simulink model "Simulink_serial_example"  (Simulink 8.8)
settings: Solver=FixedStepDiscrete  StartTime=0.0  StopTime=50  RelTol=1e-3  EnableMultiTasking=on
undefined symbols (not defined in the file or in its folder): fdesignblkfcn, gcbh, serial
libraries: instrumentlib x2
settings Model: Creator=skolak  LastModifiedBy=qhsam
settings OptimizationCC: InitFltsAndDblsToZero=on
settings DebuggingCC: SaveWithParameterizedLinksMsg=none  SignalResolutionControl=TryResolveAllWithWarning  SolverPrmCheckMsg=warning  MultiTaskDSMMsg=warning  MultiTaskCondExecSysMsg=none  StateNameClashWarn=none
settings GRTTargetCC: TargetFcnLib=ansi_tfl_tmw.mat  GeneratePreprocessorConditionals=Use local settings

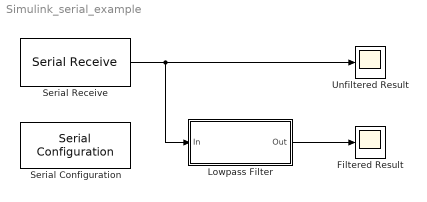
== system Simulink_serial_example ==
  Filtered Result : Scope
  Lowpass Filter : Subsystem  DialogController=fdesignblkfcn  DialogControllerArgs=DataTag1  InitFcn=fdesignblkfcn(gcbh, {'InitFcn'});  mask(Lowpass Filter){}
      mask help: Design a lowpass filter
      settings: CopyFcn=fdesignblkfcn(gcbh, {'CopyFcn'});
      mask Help: helpview(mapfilelocation('dspblks'), 'dsplowpassfilter')
      mask Display: disp('Lowpass')
  Serial Configuration : instrumentlib/Serial Configuration  Priority=-200000  ComPortMenu=COM5  ComPort=COM5  ObjConstructor=serial('COM5');  BaudRate=9600  DataBits=8  Parity=none  StopBits=1  FlowControl=none  Timeout=10  ByteOrder=LittleEndian
  Serial Receive : instrumentlib/Serial Receive  ComPortMenu=COM5  ComPort=COM5  ObjConstructor=serial('COM5');  Terminator=<none>  DataSize=[1 1]  DataType=uint8  EnableBlockingMode=on  ActionDataUnavailable=Output last received value  CustomValue=0  SampleTime=0.01
  Unfiltered Result : Scope
  wires:
  Lowpass Filter/1(Out) -> Filtered Result/1
  Serial Receive/1 -> Lowpass Filter/1(In), Unfiltered Result/1

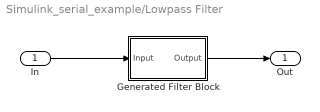
== system Simulink_serial_example/Lowpass Filter ==
  In : Inport
  Generated Filter Block : Subsystem  Tag=FilterWizardSubSystem
      settings: ErrorFcn=dspFilterRealizedInBasicElemsAlgLoopErrFcnCallback
  Out : Outport
  wires:
  In/1 -> Generated Filter Block/1(Input)
  Generated Filter Block/1(Output) -> Out/1

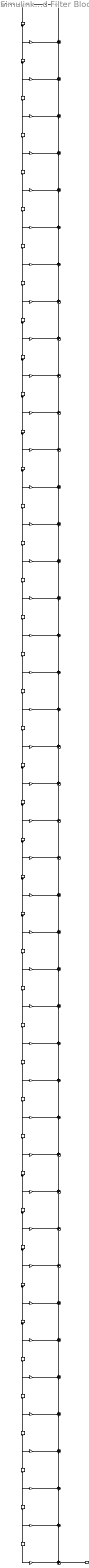
== system Simulink_serial_example/Lowpass Filter/Generated Filter Block ==
  Input : Inport
  BodyDelay{2..43} (42 alike) : Delay  DelayLength=1  InitialCondition=0  InputProcessing=Inherited
  BodyLSum{2..43} (42 alike) : Sum  Inputs=++|  RndMeth=Nearest  SaturateOnIntegerOverflow=on  OutDataTypeStr=Inherit: Same as first input
  b(1) : Gain  Gain=-0.002422873852326935  ParamDataTypeStr=double  RndMeth=Nearest  SaturateOnIntegerOverflow=on  OutDataTypeStr=Inherit: Same as input
  b(10) : Gain  Gain=-0.010121234703278952  ParamDataTypeStr=double  RndMeth=Nearest  SaturateOnIntegerOverflow=on  OutDataTypeStr=Inherit: Same as input
  b(11) : Gain  Gain=-0.018273518733782461  ParamDataTypeStr=double  RndMeth=Nearest  SaturateOnIntegerOverflow=on  OutDataTypeStr=Inherit: Same as input
  b(12) : Gain  Gain=0.011431962071777995  ParamDataTypeStr=double  RndMeth=Nearest  SaturateOnIntegerOverflow=on  OutDataTypeStr=Inherit: Same as input
  b(13) : Gain  Gain=0.026175888580407654  ParamDataTypeStr=double  RndMeth=Nearest  SaturateOnIntegerOverflow=on  OutDataTypeStr=Inherit: Same as input
  b(14) : Gain  Gain=-0.012489027835322949  ParamDataTypeStr=double  RndMeth=Nearest  SaturateOnIntegerOverflow=on  OutDataTypeStr=Inherit: Same as input
  b(15) : Gain  Gain=-0.037996623145463641  ParamDataTypeStr=double  RndMeth=Nearest  SaturateOnIntegerOverflow=on  OutDataTypeStr=Inherit: Same as input
  b(16) : Gain  Gain=0.013388945199366911  ParamDataTypeStr=double  RndMeth=Nearest  SaturateOnIntegerOverflow=on  OutDataTypeStr=Inherit: Same as input
  b(17) : Gain  Gain=0.05815546581472987  ParamDataTypeStr=double  RndMeth=Nearest  SaturateOnIntegerOverflow=on  OutDataTypeStr=Inherit: Same as input
  b(18) : Gain  Gain=-0.014048043515808944  ParamDataTypeStr=double  RndMeth=Nearest  SaturateOnIntegerOverflow=on  OutDataTypeStr=Inherit: Same as input
  b(19) : Gain  Gain=-0.10272466857882172  ParamDataTypeStr=double  RndMeth=Nearest  SaturateOnIntegerOverflow=on  OutDataTypeStr=Inherit: Same as input
  b(2) : Gain  Gain=-0.0020832449820792948  ParamDataTypeStr=double  RndMeth=Nearest  SaturateOnIntegerOverflow=on  OutDataTypeStr=Inherit: Same as input
  b(20) : Gain  Gain=0.014462275771238391  ParamDataTypeStr=double  RndMeth=Nearest  SaturateOnIntegerOverflow=on  OutDataTypeStr=Inherit: Same as input
  b(21) : Gain  Gain=0.31716649721769491  ParamDataTypeStr=double  RndMeth=Nearest  SaturateOnIntegerOverflow=on  OutDataTypeStr=Inherit: Same as input
  b(22) : Gain  Gain=0.48538764678732516  ParamDataTypeStr=double  RndMeth=Nearest  SaturateOnIntegerOverflow=on  OutDataTypeStr=Inherit: Same as input
  b(23) : Gain  Gain=0.31716649721769491  ParamDataTypeStr=double  RndMeth=Nearest  SaturateOnIntegerOverflow=on  OutDataTypeStr=Inherit: Same as input
  b(24) : Gain  Gain=0.014462275771238391  ParamDataTypeStr=double  RndMeth=Nearest  SaturateOnIntegerOverflow=on  OutDataTypeStr=Inherit: Same as input
  b(25) : Gain  Gain=-0.10272466857882172  ParamDataTypeStr=double  RndMeth=Nearest  SaturateOnIntegerOverflow=on  OutDataTypeStr=Inherit: Same as input
  b(26) : Gain  Gain=-0.014048043515808944  ParamDataTypeStr=double  RndMeth=Nearest  SaturateOnIntegerOverflow=on  OutDataTypeStr=Inherit: Same as input
  b(27) : Gain  Gain=0.05815546581472987  ParamDataTypeStr=double  RndMeth=Nearest  SaturateOnIntegerOverflow=on  OutDataTypeStr=Inherit: Same as input
  b(28) : Gain  Gain=0.013388945199366911  ParamDataTypeStr=double  RndMeth=Nearest  SaturateOnIntegerOverflow=on  OutDataTypeStr=Inherit: Same as input
  b(29) : Gain  Gain=-0.037996623145463641  ParamDataTypeStr=double  RndMeth=Nearest  SaturateOnIntegerOverflow=on  OutDataTypeStr=Inherit: Same as input
  b(3) : Gain  Gain=0.0067703446401186605  ParamDataTypeStr=double  RndMeth=Nearest  SaturateOnIntegerOverflow=on  OutDataTypeStr=Inherit: Same as input
  b(30) : Gain  Gain=-0.012489027835322949  ParamDataTypeStr=double  RndMeth=Nearest  SaturateOnIntegerOverflow=on  OutDataTypeStr=Inherit: Same as input
  b(31) : Gain  Gain=0.026175888580407654  ParamDataTypeStr=double  RndMeth=Nearest  SaturateOnIntegerOverflow=on  OutDataTypeStr=Inherit: Same as input
  b(32) : Gain  Gain=0.011431962071777995  ParamDataTypeStr=double  RndMeth=Nearest  SaturateOnIntegerOverflow=on  OutDataTypeStr=Inherit: Same as input
  b(33) : Gain  Gain=-0.018273518733782461  ParamDataTypeStr=double  RndMeth=Nearest  SaturateOnIntegerOverflow=on  OutDataTypeStr=Inherit: Same as input
  b(34) : Gain  Gain=-0.010121234703278952  ParamDataTypeStr=double  RndMeth=Nearest  SaturateOnIntegerOverflow=on  OutDataTypeStr=Inherit: Same as input
  b(35) : Gain  Gain=0.012982883808855773  ParamDataTypeStr=double  RndMeth=Nearest  SaturateOnIntegerOverflow=on  OutDataTypeStr=Inherit: Same as input
  b(36) : Gain  Gain=0.0092567976151380332  ParamDataTypeStr=double  RndMeth=Nearest  SaturateOnIntegerOverflow=on  OutDataTypeStr=Inherit: Same as input
  b(37) : Gain  Gain=-0.008401617186026885  ParamDataTypeStr=double  RndMeth=Nearest  SaturateOnIntegerOverflow=on  OutDataTypeStr=Inherit: Same as input
  b(38) : Gain  Gain=-0.0062311454141445342  ParamDataTypeStr=double  RndMeth=Nearest  SaturateOnIntegerOverflow=on  OutDataTypeStr=Inherit: Same as input
  b(39) : Gain  Gain=0.011117076081077591  ParamDataTypeStr=double  RndMeth=Nearest  SaturateOnIntegerOverflow=on  OutDataTypeStr=Inherit: Same as input
  b(4) : Gain  Gain=0.01673194542348902  ParamDataTypeStr=double  RndMeth=Nearest  SaturateOnIntegerOverflow=on  OutDataTypeStr=Inherit: Same as input
  b(40) : Gain  Gain=0.01673194542348902  ParamDataTypeStr=double  RndMeth=Nearest  SaturateOnIntegerOverflow=on  OutDataTypeStr=Inherit: Same as input
  b(41) : Gain  Gain=0.0067703446401186605  ParamDataTypeStr=double  RndMeth=Nearest  SaturateOnIntegerOverflow=on  OutDataTypeStr=Inherit: Same as input
  b(42) : Gain  Gain=-0.0020832449820792948  ParamDataTypeStr=double  RndMeth=Nearest  SaturateOnIntegerOverflow=on  OutDataTypeStr=Inherit: Same as input
  b(43) : Gain  Gain=-0.002422873852326935  ParamDataTypeStr=double  RndMeth=Nearest  SaturateOnIntegerOverflow=on  OutDataTypeStr=Inherit: Same as input
  b(5) : Gain  Gain=0.011117076081077591  ParamDataTypeStr=double  RndMeth=Nearest  SaturateOnIntegerOverflow=on  OutDataTypeStr=Inherit: Same as input
  b(6) : Gain  Gain=-0.0062311454141445342  ParamDataTypeStr=double  RndMeth=Nearest  SaturateOnIntegerOverflow=on  OutDataTypeStr=Inherit: Same as input
  b(7) : Gain  Gain=-0.008401617186026885  ParamDataTypeStr=double  RndMeth=Nearest  SaturateOnIntegerOverflow=on  OutDataTypeStr=Inherit: Same as input
  b(8) : Gain  Gain=0.0092567976151380332  ParamDataTypeStr=double  RndMeth=Nearest  SaturateOnIntegerOverflow=on  OutDataTypeStr=Inherit: Same as input
  b(9) : Gain  Gain=0.012982883808855773  ParamDataTypeStr=double  RndMeth=Nearest  SaturateOnIntegerOverflow=on  OutDataTypeStr=Inherit: Same as input
  Output : Outport
  wires:
  Input/1 -> b(1)/1, BodyDelay2/1
  b(1)/1 -> BodyLSum2/2
  BodyDelay2/1 -> b(2)/1, BodyDelay3/1
  b(2)/1 -> BodyLSum2/1
  BodyLSum2/1 -> BodyLSum3/2
  BodyDelay3/1 -> b(3)/1, BodyDelay4/1
  b(3)/1 -> BodyLSum3/1
  BodyLSum3/1 -> BodyLSum4/2
  BodyDelay4/1 -> b(4)/1, BodyDelay5/1
  b(4)/1 -> BodyLSum4/1
  BodyLSum4/1 -> BodyLSum5/2
  BodyDelay5/1 -> b(5)/1, BodyDelay6/1
  b(5)/1 -> BodyLSum5/1
  BodyLSum5/1 -> BodyLSum6/2
  BodyDelay6/1 -> b(6)/1, BodyDelay7/1
  b(6)/1 -> BodyLSum6/1
  BodyLSum6/1 -> BodyLSum7/2
  BodyDelay7/1 -> b(7)/1, BodyDelay8/1
  b(7)/1 -> BodyLSum7/1
  BodyLSum7/1 -> BodyLSum8/2
  BodyDelay8/1 -> b(8)/1, BodyDelay9/1
  b(8)/1 -> BodyLSum8/1
  BodyLSum8/1 -> BodyLSum9/2
  BodyDelay9/1 -> b(9)/1, BodyDelay10/1
  b(9)/1 -> BodyLSum9/1
  BodyLSum9/1 -> BodyLSum10/2
  BodyDelay10/1 -> b(10)/1, BodyDelay11/1
  b(10)/1 -> BodyLSum10/1
  BodyLSum10/1 -> BodyLSum11/2
  BodyDelay11/1 -> b(11)/1, BodyDelay12/1
  b(11)/1 -> BodyLSum11/1
  BodyLSum11/1 -> BodyLSum12/2
  BodyDelay12/1 -> b(12)/1, BodyDelay13/1
  b(12)/1 -> BodyLSum12/1
  BodyLSum12/1 -> BodyLSum13/2
  BodyDelay13/1 -> b(13)/1, BodyDelay14/1
  b(13)/1 -> BodyLSum13/1
  BodyLSum13/1 -> BodyLSum14/2
  BodyDelay14/1 -> b(14)/1, BodyDelay15/1
  b(14)/1 -> BodyLSum14/1
  BodyLSum14/1 -> BodyLSum15/2
  BodyDelay15/1 -> b(15)/1, BodyDelay16/1
  b(15)/1 -> BodyLSum15/1
  BodyLSum15/1 -> BodyLSum16/2
  BodyDelay16/1 -> b(16)/1, BodyDelay17/1
  b(16)/1 -> BodyLSum16/1
  BodyLSum16/1 -> BodyLSum17/2
  BodyDelay17/1 -> b(17)/1, BodyDelay18/1
  b(17)/1 -> BodyLSum17/1
  BodyLSum17/1 -> BodyLSum18/2
  BodyDelay18/1 -> b(18)/1, BodyDelay19/1
  b(18)/1 -> BodyLSum18/1
  BodyLSum18/1 -> BodyLSum19/2
  BodyDelay19/1 -> b(19)/1, BodyDelay20/1
  b(19)/1 -> BodyLSum19/1
  BodyLSum19/1 -> BodyLSum20/2
  BodyDelay20/1 -> b(20)/1, BodyDelay21/1
  b(20)/1 -> BodyLSum20/1
  BodyLSum20/1 -> BodyLSum21/2
  BodyDelay21/1 -> b(21)/1, BodyDelay22/1
  b(21)/1 -> BodyLSum21/1
  BodyLSum21/1 -> BodyLSum22/2
  BodyDelay22/1 -> b(22)/1, BodyDelay23/1
  b(22)/1 -> BodyLSum22/1
  BodyLSum22/1 -> BodyLSum23/2
  BodyDelay23/1 -> b(23)/1, BodyDelay24/1
  b(23)/1 -> BodyLSum23/1
  BodyLSum23/1 -> BodyLSum24/2
  BodyDelay24/1 -> b(24)/1, BodyDelay25/1
  b(24)/1 -> BodyLSum24/1
  BodyLSum24/1 -> BodyLSum25/2
  BodyDelay25/1 -> b(25)/1, BodyDelay26/1
  b(25)/1 -> BodyLSum25/1
  BodyLSum25/1 -> BodyLSum26/2
  BodyDelay26/1 -> b(26)/1, BodyDelay27/1
  b(26)/1 -> BodyLSum26/1
  BodyLSum26/1 -> BodyLSum27/2
  BodyDelay27/1 -> b(27)/1, BodyDelay28/1
  b(27)/1 -> BodyLSum27/1
  BodyLSum27/1 -> BodyLSum28/2
  BodyDelay28/1 -> b(28)/1, BodyDelay29/1
  b(28)/1 -> BodyLSum28/1
  BodyLSum28/1 -> BodyLSum29/2
  BodyDelay29/1 -> b(29)/1, BodyDelay30/1
  b(29)/1 -> BodyLSum29/1
  BodyLSum29/1 -> BodyLSum30/2
  BodyDelay30/1 -> b(30)/1, BodyDelay31/1
  b(30)/1 -> BodyLSum30/1
  BodyLSum30/1 -> BodyLSum31/2
  BodyDelay31/1 -> b(31)/1, BodyDelay32/1
  b(31)/1 -> BodyLSum31/1
  BodyLSum31/1 -> BodyLSum32/2
  BodyDelay32/1 -> b(32)/1, BodyDelay33/1
  b(32)/1 -> BodyLSum32/1
  BodyLSum32/1 -> BodyLSum33/2
  BodyDelay33/1 -> b(33)/1, BodyDelay34/1
  b(33)/1 -> BodyLSum33/1
  BodyLSum33/1 -> BodyLSum34/2
  BodyDelay34/1 -> b(34)/1, BodyDelay35/1
  b(34)/1 -> BodyLSum34/1
  BodyLSum34/1 -> BodyLSum35/2
  BodyDelay35/1 -> b(35)/1, BodyDelay36/1
  b(35)/1 -> BodyLSum35/1
  BodyLSum35/1 -> BodyLSum36/2
  BodyDelay36/1 -> b(36)/1, BodyDelay37/1
  b(36)/1 -> BodyLSum36/1
  BodyLSum36/1 -> BodyLSum37/2
  BodyDelay37/1 -> b(37)/1, BodyDelay38/1
  b(37)/1 -> BodyLSum37/1
  BodyLSum37/1 -> BodyLSum38/2
  BodyDelay38/1 -> b(38)/1, BodyDelay39/1
  b(38)/1 -> BodyLSum38/1
  BodyLSum38/1 -> BodyLSum39/2
  BodyDelay39/1 -> b(39)/1, BodyDelay40/1
  b(39)/1 -> BodyLSum39/1
  BodyLSum39/1 -> BodyLSum40/2
  BodyDelay40/1 -> b(40)/1, BodyDelay41/1
  b(40)/1 -> BodyLSum40/1
  BodyLSum40/1 -> BodyLSum41/2
  BodyDelay41/1 -> b(41)/1, BodyDelay42/1
  b(41)/1 -> BodyLSum41/1
  BodyLSum41/1 -> BodyLSum42/2
  BodyDelay42/1 -> b(42)/1, BodyDelay43/1
  b(42)/1 -> BodyLSum42/1
  BodyLSum42/1 -> BodyLSum43/1
  BodyDelay43/1 -> b(43)/1
  b(43)/1 -> BodyLSum43/2
  BodyLSum43/1 -> Output/1
